simulink model "first"  (R2016a)
settings: Solver=VariableStepAuto  StartTime=0.0  StopTime=10.0  RelTol=1e-3
settings Model: Creator=kypis  LastModifiedBy=kypis

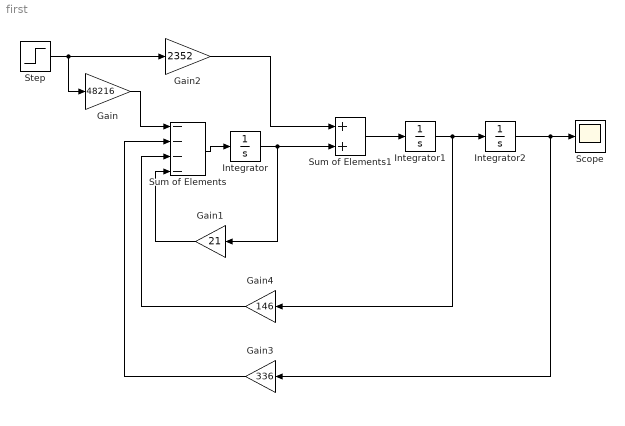
== system first ==
  Gain : Gain  Gain=48216
  Gain1 : Gain  Gain=21
  Gain2 : Gain  Gain=2352
  Gain3 : Gain  Gain=336
  Gain4 : Gain  Gain=146
  Integrator : Integrator
  Integrator1 : Integrator
  Integrator2 : Integrator
  Scope : Scope
  Step : Step  Time=0  SampleTime=0
  Sum of Elements : Sum  Inputs=----
  Sum of Elements1 : Sum
  wires:
  Sum of Elements/1 -> Integrator/1
  Step/1 -> Gain/1, Gain2/1
  Gain/1 -> Sum of Elements/1
  Integrator/1 -> Sum of Elements1/2, Gain1/1
  Gain1/1 -> Sum of Elements/4
  Sum of Elements1/1 -> Integrator1/1
  Integrator1/1 -> Gain4/1, Integrator2/1
  Gain2/1 -> Sum of Elements1/1
  Integrator2/1 -> Gain3/1, Scope/1
  Gain4/1 -> Sum of Elements/3
  Gain3/1 -> Sum of Elements/2
